simulink model "lookupTableDynamic_TestGen39"  (R2017b)
settings: Solver=FixedStepDiscrete  StartTime=0.0  StopTime=10.0  RelTol=1e-3
libraries: simulink x1
settings Model: Creator=ktrinh  LastModifiedBy=ktrinh
settings DebuggingCC: ParameterOverflowMsg=none

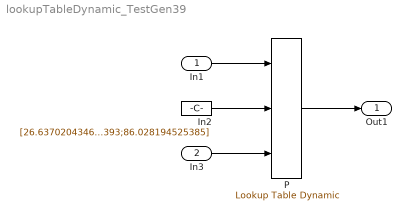
== system lookupTableDynamic_TestGen39 ==
  In1 : Inport  OutMin=24.637  OutMax=88  OutDataTypeStr=int32  PortDimensions=[2,3]
  In3 : Inport  Port=2  PortDimensions=5
  In2 : Constant  Value=[26.6370204346697;44.7901520998838;57.5475641030585;62.6385315053393;86.028194525385]  OutDataTypeStr=int32
  P : simulink/Lookup Tables/Lookup Table Dynamic  LookUpMeth=Use Input Above  OutDataType=fixdt('int8')  OutScaling=[]  OutputDataTypeScalingMode=Specify via dialog  OutDataTypeStr=int8  RndMeth=Round  DoSatur=on
      settings: SourceProductName=Simulink
  Out1 : Outport
  wires:
  In1/1 -> P/1
  In2/1 -> P/2
  In3/1 -> P/3
  P/1 -> Out1/1
